simulink model "arwSimulation"  (R2019b)
settings: Solver=VariableStepAuto  StartTime=0.0  StopTime=10  RelTol=1e-3
values from neighbouring files (symbols this model uses):
  m_nom = 1    [SISO_x.m]    (also in basicSISO_x.m; basicSISO_y.m; loadSystemVariables.m)
  s = qctrl(0,[],1)    [SISO_phi.m]    (also in SISO_x.m; basicSISO_phi.m; basicSISO_x.m; basicSISO_y.m)
  tau = 0.075    [loadSystemVariables.m]
libraries: cstblocks x3
settings Model: Creator=Iftah  LastModifiedBy=Iftah
settings SolverCC: ZeroCrossAlgorithm=Adaptive
settings DebuggingCC: IgnoredZcDiagnostic=none

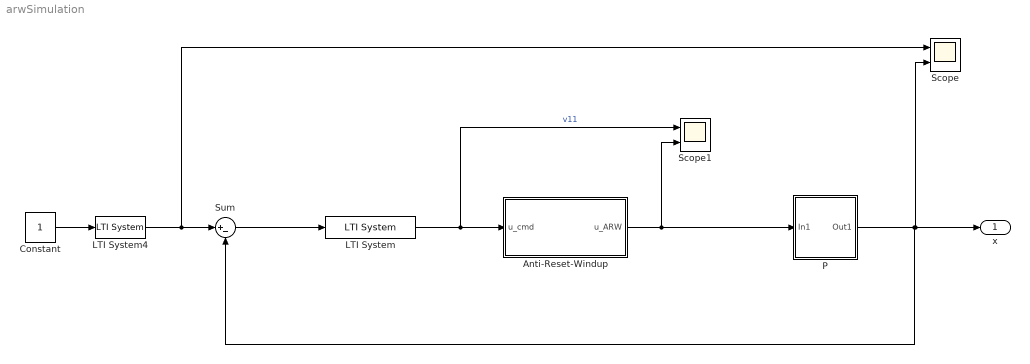
== system arwSimulation ==
  Anti-Reset-Windup : Subsystem
  Constant : Constant
  LTI System : cstblocks/LTI System  sys=Gv  IC=[]
  LTI System4 : cstblocks/LTI System  sys=Fv  IC=[]
  P : Subsystem
  Scope : Scope  NumInputPorts=2
  Scope1 : Scope  NumInputPorts=2
  Sum : Sum  Inputs=|+-
  x : Outport
  wires:
  LTI System/1 -> Anti-Reset-Windup/1(u_cmd), Scope1/1  "v11"
  P/1(Out1) -> Sum/2, Scope/2, x/1
  Sum/1 -> LTI System/1
  Constant/1 -> LTI System4/1
  LTI System4/1 -> Sum/1, Scope/1
  Anti-Reset-Windup/1(u_ARW) -> Scope1/2, P/1(In1)

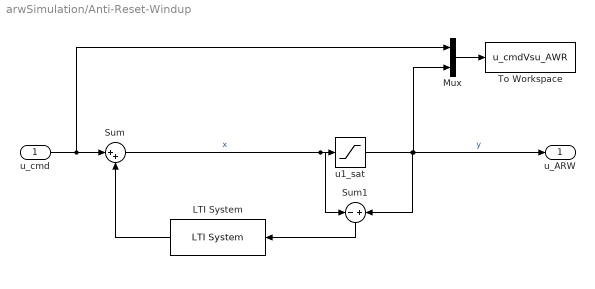
== system arwSimulation/Anti-Reset-Windup ==
  u_cmd : Inport
  LTI System : cstblocks/LTI System  sys=tf(s)/(tf(s^2)+0.1)  IC=[]
  Mux : Mux  Inputs=2
  Sum : Sum  Inputs=|++
  Sum1 : Sum  Inputs=-|+
  To Workspace : ToWorkspace  VariableName=u_cmdVsu_AWR  SaveFormat=Timeseries  SampleTime=-1
  u1_sat : Saturate  UpperLimit=80  LowerLimit=-80
  u_ARW : Outport
  wires:
  u_cmd/1 -> Mux/1, Sum/1
  u1_sat/1 -> Sum1/2, Mux/2, u_ARW/1  "y"
  Sum/1 -> Sum1/1, u1_sat/1  "x"
  Sum1/1 -> LTI System/1
  LTI System/1 -> Sum/2
  Mux/1 -> To Workspace/1

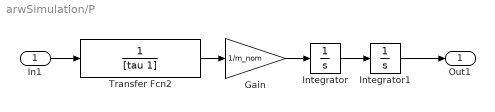
== system arwSimulation/P ==
  In1 : Inport
  Gain : Gain  Gain=1/m_nom
  Integrator : Integrator
  Integrator1 : Integrator
  Transfer Fcn2 : TransferFcn  Denominator=[tau 1]
  Out1 : Outport
  wires:
  Gain/1 -> Integrator/1
  In1/1 -> Transfer Fcn2/1
  Integrator/1 -> Integrator1/1
  Integrator1/1 -> Out1/1
  Transfer Fcn2/1 -> Gain/1
